simulink model "AMPC_TEST"  (R2020a)
settings: Solver=FixedStepAuto  StartTime=0.0  StopTime=10.0  FixedStep=Ts  RelTol=1e-3
undefined symbols (not defined in the file or in its folder): Ts
libraries: mympclib x2, Meldas_library x1
settings Model: Creator=kohei  LastModifiedBy=kohei
settings OptimizationCC: DefaultParameterBehavior=Inlined  EnhancedBackFolding=on  PassReuseOutputArgsAs=Individual arguments  ZeroExternalMemoryAtStartup=off  ZeroInternalMemoryAtStartup=off  OptimizeBlockOrder=speed  DifferentSizesBufferReuse=on  OptimizationCustomize=off  EfficientTunableParamExpr=on
settings DebuggingCC: ParameterTunabilityLossMsg=error  BusObjectLabelMismatch=error
settings SFSimCC: MATLABDynamicMemAlloc=off
settings RTWCC: SystemTargetFile=ert.tlc  TemplateMakefile=ert_default_tmf  GenerateReport=on  IncludeHyperlinkInReport=on  LaunchReport=on  GenerateTraceInfo=on  GenerateTraceReport=on  GenerateTraceReportSl=on  GenerateTraceReportSf=on  GenerateTraceReportEml=on
settings CodeAppCC: ForceParamTrailComments=on  IgnoreCustomStorageClasses=off  OperatorAnnotations=on  SimulinkDataObjDesc=on  SFDataObjDesc=on  InsertBlockDesc=on
settings ERTTargetCC: TargetLangStandard=C99 (ISO)  GenerateSampleERTMain=on  InlinedParameterPlacement=NonHierarchical  ERTCustomFileTemplate=example_file_process.tlc

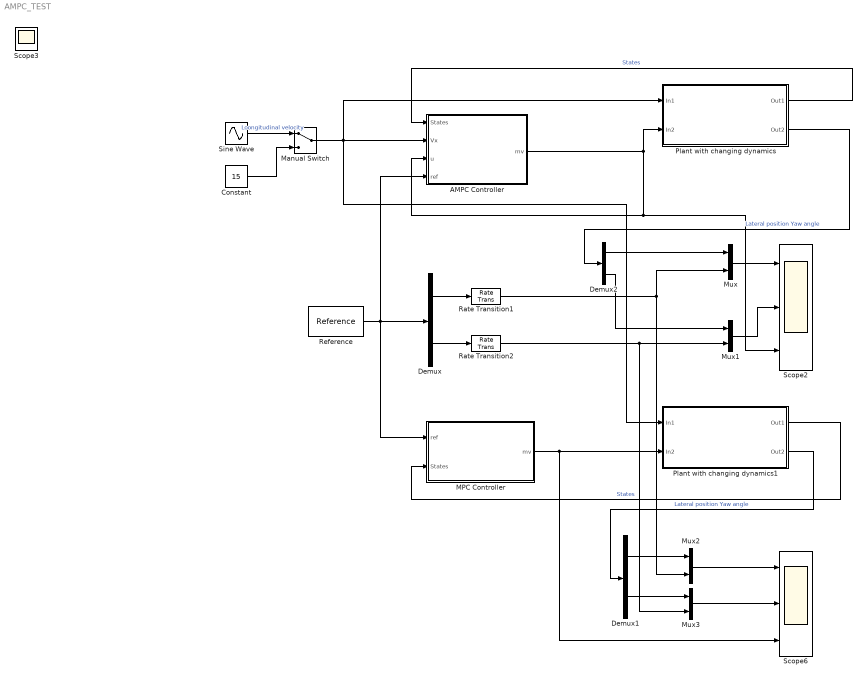
== system AMPC_TEST ==
  AMPC Controller : Subsystem
  Constant : Constant  Value=15
  Demux : Demux  Outputs=2
  Demux1 : Demux  Outputs=2
  Demux2 : Demux  Outputs=2
  MPC Controller : Subsystem
  Manual Switch : ManualSwitch
  Mux{,1..3} (4 alike) : Mux  Inputs=2
  Plant with changing dynamics : Subsystem
      mask Display: image('car.jpg');
  Plant with changing dynamics1 : Subsystem
      mask Display: image('car.jpg');
  Rate Transition1 : RateTransition  OutPortSampleTime=0
  Rate Transition2 : RateTransition  OutPortSampleTime=0
  Reference : Meldas_library/Reference  SystemSampleTime=-1  Latency=0  AutoFrameSizeCalculation=off
  Scope2 : Scope  NumInputPorts=3
  Scope6 : Scope  NumInputPorts=3
  Sine Wave : Sin  Amplitude=50  Bias=15  Frequency=0.1  SampleTime=0
  Scope3 : Scope
  wires:
  Plant with changing dynamics/2(Out2) -> Demux2/1  "Lateral position Yaw angle"
  Mux1/1 -> Scope2/2
  Mux/1 -> Scope2/1
  Demux2/2 -> Mux1/1
  Rate Transition2/1 -> Mux1/2, Mux3/2
  Demux2/1 -> Mux/1
  Rate Transition1/1 -> Mux2/2, Mux/2
  Mux3/1 -> Scope6/2
  Mux2/1 -> Scope6/1
  Demux1/1 -> Mux2/1
  Demux1/2 -> Mux3/1
  Plant with changing dynamics1/2(Out2) -> Demux1/1  "Lateral position Yaw angle"
  Sine Wave/1 -> Manual Switch/1  "Loongitudinal velocity"
  Manual Switch/1 -> Plant with changing dynamics/1(In1), Plant with changing dynamics1/1(In1), AMPC Controller/2(Vx)
  Constant/1 -> Manual Switch/2
  AMPC Controller/1(mv) -> Scope2/3, AMPC Controller/3(u), Plant with changing dynamics/2(In2)
  Plant with changing dynamics/1(Out1) -> AMPC Controller/1(States)  "States"
  MPC Controller/1(mv) -> Plant with changing dynamics1/2(In2), Scope6/3
  Plant with changing dynamics1/1(Out1) -> MPC Controller/2(States)  "States"
  Demux/1 -> Rate Transition1/1
  Demux/2 -> Rate Transition2/1
  Reference/1 -> MPC Controller/1(ref), AMPC Controller/4(ref), Demux/1

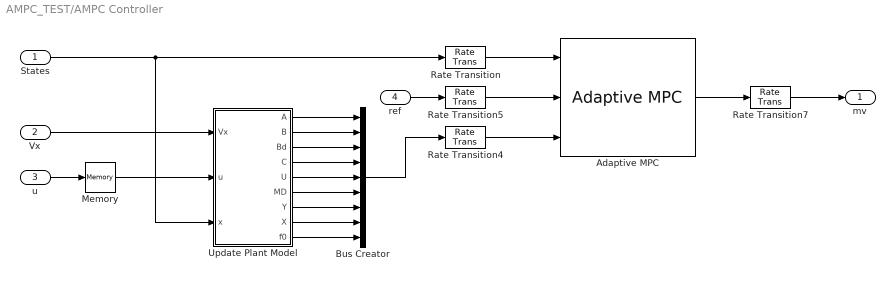
== system AMPC_TEST/AMPC Controller ==
  States : Inport
  Vx : Inport  Port=2
  u : Inport  Port=3
  ref : Inport  Port=4
  Adaptive MPC : mympclib/Adaptive MPC  params=params  numState=4  numRef=2  numMV=1  Ts=Ts  enableDist=off  numDist=1  enableSlack=off  enableStatus=off  enableMVseq=off
      settings: SourceProductName=My MPC Library
  Bus Creator : BusCreator  Inputs=9  OutDataTypeStr=Bus: sysBus
  Memory : Memory
  Rate Transition : RateTransition  OutPortSampleTime=Ts
  Rate Transition4 : RateTransition  OutPortSampleTime=Ts
  Rate Transition5 : RateTransition  OutPortSampleTime=Ts
  Rate Transition7 : RateTransition  OutPortSampleTime=0
  Update Plant Model : MATLAB Function  TreatAsAtomicUnit=on
  mv : Outport
  wires:
  Adaptive MPC/1 -> Rate Transition7/1
  Bus Creator/1 -> Rate Transition4/1
  Rate Transition5/1 -> Adaptive MPC/2
  States/1 -> Update Plant Model/3(x), Rate Transition/1
  Memory/1 -> Update Plant Model/2(u)
  Rate Transition7/1 -> mv/1
  Vx/1 -> Update Plant Model/1(Vx)
  ref/1 -> Rate Transition5/1
  u/1 -> Memory/1
  Update Plant Model/1(A) -> Bus Creator/1
  Update Plant Model/2(B) -> Bus Creator/2
  Update Plant Model/3(Bd) -> Bus Creator/3
  Update Plant Model/4(C) -> Bus Creator/4
  Update Plant Model/5(U) -> Bus Creator/5
  Update Plant Model/6(MD) -> Bus Creator/6
  Update Plant Model/7(Y) -> Bus Creator/7
  Update Plant Model/8(X) -> Bus Creator/8
  Update Plant Model/9(f0) -> Bus Creator/9
  Rate Transition/1 -> Adaptive MPC/1
  Rate Transition4/1 -> Adaptive MPC/3

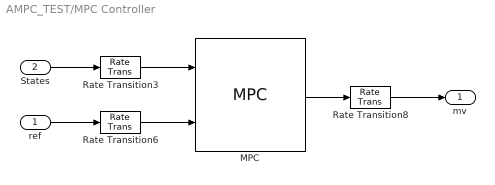
== system AMPC_TEST/MPC Controller ==
  ref : Inport
  States : Inport  Port=2
  MPC : mympclib/MPC  params=params  sysm=sysm  numState=4  numRef=2  numMV=1  Ts=Ts  enableDist=off  numDist=1  enableSlack=off  enableStatus=off  enableMVseq=off
      settings: SourceProductName=My MPC Library
  Rate Transition3 : RateTransition  OutPortSampleTime=Ts
  Rate Transition6 : RateTransition  OutPortSampleTime=Ts
  Rate Transition8 : RateTransition  OutPortSampleTime=0
  mv : Outport
  wires:
  MPC/1 -> Rate Transition8/1
  ref/1 -> Rate Transition6/1
  States/1 -> Rate Transition3/1
  Rate Transition8/1 -> mv/1
  Rate Transition3/1 -> MPC/1
  Rate Transition6/1 -> MPC/2

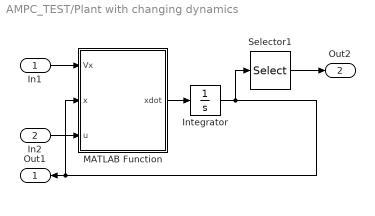
== system AMPC_TEST/Plant with changing dynamics ==
  In1 : Inport
  In2 : Inport  Port=2
  Integrator : Integrator
  MATLAB Function : MATLAB Function  TreatAsAtomicUnit=on
  Selector1 : Selector  InputPortWidth=4  IndexOptions=Index vector (dialog)  Indices=[4 2]  OutputSizes=1
  Out1 : Outport  VectorParamsAs1DForOutWhenUnconnected=off
  Out2 : Outport  Port=2  VectorParamsAs1DForOutWhenUnconnected=off
  wires:
  In2/1 -> MATLAB Function/3(u)
  In1/1 -> MATLAB Function/1(Vx)
  Integrator/1 -> Selector1/1, MATLAB Function/2(x), Out1/1
  MATLAB Function/1(xdot) -> Integrator/1
  Selector1/1 -> Out2/1

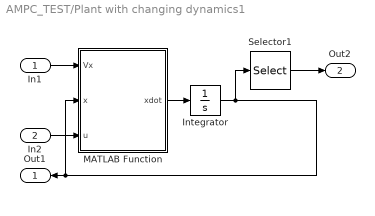
== system AMPC_TEST/Plant with changing dynamics1 ==
  In1 : Inport
  In2 : Inport  Port=2
  Integrator : Integrator
  MATLAB Function : MATLAB Function  TreatAsAtomicUnit=on
  Selector1 : Selector  InputPortWidth=4  IndexOptions=Index vector (dialog)  Indices=[4 2]  OutputSizes=1
  Out1 : Outport  VectorParamsAs1DForOutWhenUnconnected=off
  Out2 : Outport  Port=2  VectorParamsAs1DForOutWhenUnconnected=off
  wires:
  Selector1/1 -> Out2/1
  MATLAB Function/1(xdot) -> Integrator/1
  Integrator/1 -> Out1/1, MATLAB Function/2(x), Selector1/1
  In1/1 -> MATLAB Function/1(Vx)
  In2/1 -> MATLAB Function/3(u)

== matlab function AMPC_TEST/Plant with changing dynamics/MATLAB Function ==
  data: Vx input; x input size=[4,1]; u input; xdot output size=[4,1]
function xdot = fcn(Vx,x,u)

% Model parameters
m = 1575;
Iz = 2875;
lf = 1.2;
lr = 1.6;
Cf = 19000;
Cr = 33000;

% Continuous-time model
A = [-(2*Cf+2*Cr)/m/Vx, 0, -Vx-(2*Cf*lf-2*Cr*lr)/m/Vx, 0;
     0, 0, 1, 0;
     -(2*Cf*lf-2*Cr*lr)/Iz/Vx, 0, -(2*Cf*lf^2+2*Cr*lr^2)/Iz/Vx, 0;
     1, Vx, 0, 0];
B = [2*Cf/m 0 2*Cf*lf/Iz 0]';   
C = [0 0 0 1; 0 1 0 0];
D = zeros(2,1);
xdot = A*x + B*u;
%y = C*x + D*u;

== matlab function AMPC_TEST/AMPC Controller/Update Plant Model ==
  data: Vx input; u input; A output size=[4,4]; x input size=[4,1]; B output size=[4,1]; Bd output size=[4,1]; C output size=[2,4]; U output size=1; MD output size=1; Y output size=[2,1]; X output size=[4,1]; f0 output size=[4,1]; Ts parameter
function [A,B,Bd,C,U,MD,Y,X,f0] = fcn(Vx,u,x,Ts)
[A,B,Bd,C,U,MD,Y,X,f0] = calcPlantModelDT(Ts,Vx,u,x);

== matlab function AMPC_TEST/Plant with changing dynamics1/MATLAB Function ==
  data: Vx input; x input size=[4,1]; u input; xdot output size=[4,1]
function xdot = fcn(Vx,x,u)

% Model parameters
m = 1575;
Iz = 2875;
lf = 1.2;
lr = 1.6;
Cf = 19000;
Cr = 33000;

% Continuous-time model
A = [-(2*Cf+2*Cr)/m/Vx, 0, -Vx-(2*Cf*lf-2*Cr*lr)/m/Vx, 0;
     0, 0, 1, 0;
     -(2*Cf*lf-2*Cr*lr)/Iz/Vx, 0, -(2*Cf*lf^2+2*Cr*lr^2)/Iz/Vx, 0;
     1, Vx, 0, 0];
B = [2*Cf/m 0 2*Cf*lf/Iz 0]';   
C = [0 0 0 1; 0 1 0 0];
D = zeros(2,1);
xdot = A*x + B*u;
%y = C*x + D*u;
